simulink model "slexResettableConfigurationExample"  (R2019b)
settings: Solver=ode45  StartTime=0.0  StopTime=10  MaxStep=0.1  RelTol=1e-3  AbsTol=1e-6
undefined symbols (not defined in the file): DiscIntNeverNeededParam
Description:
  | Discrete and Continuous Resettable Subsystems
  | 
  | This example shows the comparison between behaviors of discrete and continuous resettable subsystems.
  | After running the simulation, the two scopes show the results for the discrete resettable
  | subsystem (top scope), and continuous enabled subsystems (bottom scope).
settings Model: ExtModeTrigMode=oneshot  ExtModeArmWhenConnect=off  ExtModeAutoUpdateStatusClock=off  Creator=The MathWorks, Inc.  LastModifiedBy=bhisma
settings SolverCC: AutoScaleAbsTol=off
settings DataIOCC: ExternalInput=[]  InitialState=[]  SaveFormat=StructureWithTime
settings OptimizationCC: BlockReduction=off  BooleanDataType=off  ExpressionDepthLimit=2147483647  InitFltsAndDblsToZero=on  LifeSpan=inf
settings DebuggingCC: SaveWithParameterizedLinksMsg=none  SignalResolutionControl=TryResolveAllWithWarning  MultiTaskDSMMsg=warning  MultiTaskCondExecSysMsg=none  FcnCallInpInsideContextMsg=warning  AllowSymbolicDim=off  StateNameClashWarn=warning  SFUnexpectedBacktrackingDiag=warning  SFNoUnconditionalDefaultTransitionDiag=warning  SFExecutionAtInitializationDiag=none  ArithmeticOperatorsInVariantConditions=warning
settings HardwareCC: ProdBitPerPointer=32  ProdBitPerSizeT=32  ProdBitPerPtrDiffT=32  ProdLargestAtomicFloat=None  ProdIntDivRoundTo=Undefined  ProdEndianess=Unspecified  ProdWordSize=32  ProdHWDeviceType=32-bit Generic  TargetUnknown=on
settings ModelReferenceCC: PropagateSignalLabelsOutOfModel=off
settings SFSimCC: SimUseLocalCustomCode=off  CustomCodeUndefinedFunction=UseInterfaceOnly
settings RTWCC: RTWUseLocalCustomCode=off
settings CodeAppCC: StateflowObjectComments=on
settings GRTTargetCC: TargetFcnLib=ansi_tfl_tmw.mat  TargetLangStandard=C89/C90 (ANSI)  GeneratePreprocessorConditionals=Disable all  CombineOutputUpdateFcns=off  GRTInterface=on
settings ConfigComp: CovMetricSettings=dw  CovHtmlReporting=on  CovSaveCumulativeToWorkspaceVar=on  CovSaveSingleToWorkspaceVar=on  CovExternalEMLEnable=off  CovSFcnEnable=off
settings SimscapeCC: SimscapeNormalizeSystem=off
settings ConfigurationSet: Description=SimMechanics 2G

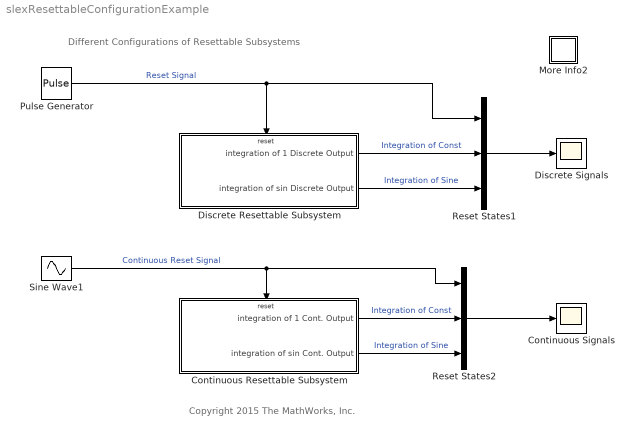
== system slexResettableConfigurationExample ==
  note: Different Configurations of Resettable Subsystems
  note: Copyright 2015 The MathWorks, Inc.
  Continuous Signals : Scope
      settings: StartFcn=open_system(gcbh)
  Continuous Resettable Subsystem : Subsystem
  Discrete Signals : Scope
      settings: StartFcn=open_system(gcbh)
  Discrete Resettable Subsystem : Subsystem
  More Info2 : Subsystem
      settings: OpenFcn=showdemo(bdroot(gcs))
      mask Display: disp('?')
  Pulse Generator : DiscretePulseGenerator  Period=40  PulseWidth=20  SampleTime=.1
  Reset States1 : Mux  Inputs=3
  Reset States2 : Mux  Inputs=3
  Sine Wave1 : Sin  Frequency=pi  SampleTime=0
  wires:
  Discrete Resettable Subsystem/1(integration of 1 Discrete Output) -> Reset States1/2  "Integration of Const"
  Discrete Resettable Subsystem/2(integration of sin Discrete Output) -> Reset States1/3  "Integration of Sine"
  Pulse Generator/1 -> Discrete Resettable Subsystem/Reset, Reset States1/1  "Reset Signal"
  Reset States1/1 -> Discrete Signals/1
  Continuous Resettable Subsystem/1(integration of 1 Cont. Output) -> Reset States2/2  "Integration of Const"
  Reset States2/1 -> Continuous Signals/1
  Sine Wave1/1 -> Reset States2/1, Continuous Resettable Subsystem/Reset  "Continuous Reset Signal"
  Continuous Resettable Subsystem/2(integration of sin Cont. Output) -> Reset States2/3  "Integration of Sine"

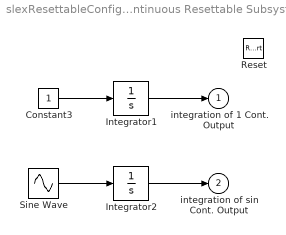
== system slexResettableConfigurationExample/Continuous Resettable Subsystem ==
  Reset : ResetPort  DisableCoverage=on
  Constant3 : Constant
  Integrator1 : Integrator
  Integrator2 : Integrator
  Sine Wave : Sin  SampleTime=0
  integration of 1 Cont. Output : Outport  InitialOutput=0  VectorParamsAs1DForOutWhenUnconnected=off
  integration of sin Cont. Output : Outport  Port=2  OutputWhenDisabled=reset  InitialOutput=0  VectorParamsAs1DForOutWhenUnconnected=off
  wires:
  Constant3/1 -> Integrator1/1
  Integrator1/1 -> integration of 1 Cont. Output/1
  Sine Wave/1 -> Integrator2/1
  Integrator2/1 -> integration of sin Cont. Output/1

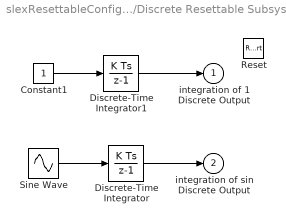
== system slexResettableConfigurationExample/Discrete Resettable Subsystem ==
  Reset : ResetPort  DisableCoverage=on  ResetTriggerType=either
  Constant1 : Constant  SampleTime=.1
  Discrete-Time Integrator : DiscreteIntegrator  SampleTime=-1  ICPrevOutput=DiscIntNeverNeededParam  ICPrevScaledInput=DiscIntNeverNeededParam
  Discrete-Time Integrator1 : DiscreteIntegrator  SampleTime=-1  ICPrevOutput=DiscIntNeverNeededParam  ICPrevScaledInput=DiscIntNeverNeededParam
  Sine Wave : Sin  SampleTime=.1
  integration of 1 Discrete Output : Outport  InitialOutput=0  VectorParamsAs1DForOutWhenUnconnected=off
  integration of sin Discrete Output : Outport  Port=2  OutputWhenDisabled=reset  InitialOutput=0  VectorParamsAs1DForOutWhenUnconnected=off
  wires:
  Discrete-Time Integrator/1 -> integration of sin Discrete Output/1
  Sine Wave/1 -> Discrete-Time Integrator/1
  Discrete-Time Integrator1/1 -> integration of 1 Discrete Output/1
  Constant1/1 -> Discrete-Time Integrator1/1

== system slexResettableConfigurationExample/More Info2 ==
